simulink model "mu_t_2021b_temp"  (R2023b)
settings: Solver=VariableStepAuto  StartTime=0.0  StopTime=120  FixedStep=0.01  RelTol=1e-3
InitFcn:
  | %rho_0t=[0.29;0.29;0.29]; %m
  | %V_0t=[-0.001;-0.001;0];%[-0.0005;-0.0005;0];
  | %w_t=[0;0;-0.002];
  | 
  | 
  | %rho_0t=[0.3;0.3;0.2]; %m
  | %V_0t=[-0.001;-0.001;0];%[-0.0005;-0.0005;0];
  | %w_t=[0;0;-0.001];
values from neighbouring files (symbols this model uses):
  g_cm = zeros(4,4,n)    [Initiate_KUKA_inv.m]    (also in KUKA_Main.m)
  iota0 = eye(6,6)    [Initiate_KUKA_inv.m]    (also in KUKA_Main.m)
  K_d = 10*[1.3*eye(3) zeros(3);zeros(3) 0.8*eye(3)]    [Initiate_FQ.m]    (also in Initiate_KUKA_inv.m = 5*[0.7*eye(3) zeros(3);zeros(3) 0.5*eye(3)]; KUKA_Main.m = 50*[0.7*eye(3) zeros(3);zeros(3) 0.5*eye(3)])
  K_i = 5*[0.1*eye(3) zeros(3);zeros(3) 0.01*eye(3)]    [Initiate_FQ.m]    (also in Initiate_KUKA_inv.m = 5*[0.01*eye(3) zeros(3);zeros(3) 0.001*eye(3)]; KUKA_Main.m = 50*[0.01*eye(3) zeros(3);zeros(3) 0.001*eye(3)])
  K_p = 100*[0.1 0 0 0 0 0;0 0.1 0 0 0 0; 0 0 0.1 0 0 0; 0 0 0 0.01 0 0 ... (first row only)    [Initiate_FQ.m]    (also in Initiate_KUKA_inv.m = 5*[0.1 0 0 0 0 0;0 0.1 0 0 0 0; 0 0 0.1 0 0 0; 0 0 0 0.01 0 ; KUKA_Main.m = 50*[0.1 0 0 0 0 0;0 0.1 0 0 0 0; 0 0 0.1 0 0 0; 0 0 0 0.01 0)
  K_w = 200*eye(7)    [Initiate_FQ.m]
  K_wd = 2*eye(7)    [Initiate_FQ.m]
  M0 = M_temp.M0.data(:,:,1)    [Initiate_FQ.m]    (also in KUKA_Main.m)
  m0 = robot.Bodies{1,n+1}.Mass    [Initiate_KUKA_inv.m]    (also in KUKA_Main.m)
  m0_frak = diag_M(1:6,1:6)    [Initiate_KUKA_inv.m]
  M0m = M_temp.M0m.data(:,:,1)    [Initiate_FQ.m]    (also in KUKA_Main.m)
  m_diag = diag_M(7:end,7:end)    [Initiate_KUKA_inv.m]
  M_t = (((Adjoint(g_It))'\M_t_body)/(Adjoint(g_It)))    [Initiate_FQ.m]    (also in Initiate_KUKA_inv.m = [eye(3)*mt zeros(3); zeros(3) eye(3)*80]; KUKA_Main.m = [eye(3)*mt zeros(3); zeros(3) eye(3)*80])
  Mm = simplify(transpose(Xi_m)*transpose(Lm)*diagM*Lm*Xi_m)    [KUKA_Main.m]
  mm = zeros(1,n)    [Initiate_KUKA_inv.m]    (also in KUKA_Main.m)
  mu = P0    [Initiate_FQ.m]    (also in Initiate_KUKA_inv.m = zeros(6,1); KUKA_Main.m = P)
  mu_t = inv((Adjoint(g_It))')*M_t_body*[V_It;w_t]    [Initiate_FQ.m]    (also in Initiate_KUKA_inv.m = M_t*[V_0t;w_t]; KUKA_Main.m = M_t*[V_0t;w_t])
  q_dot_m = [0;0;0;0;0;0;0]    [Initiate_FQ.m]    (also in Initiate_KUKA_inv.m; KUKA_Main.m = [qdot1;qdot2;qdot3;qdot4;qdot5;qdot6;qdot7])
  q_m = [0.2;1.2;0.3;2.5;0.5;1.5;0.6]    [Initiate_FQ.m]    (also in Initiate_KUKA_inv.m = [0;0;0;0;0;0;0]; KUKA_Main.m = [q_m1;q_m2;q_m3;q_m4;q_m5;q_m6;q_m7])
  rho_It = [-0.3;-0.3;-0.1]    [Initiate_FQ.m]
  sc_size = 1    [Initiate_KUKA_inv.m]    (also in KUKA_Main.m)
  V_I0 = [-0.0001;-0.0001;0.0;-0.001;0.001;0.002]    [Initiate_FQ.m]    (also in Initiate_KUKA_inv.m = [0;0;0;0;0;0]; KUKA_Main.m = [0;0;0;0;0;0])
  V_It = 0.1.*[0.01;0.01;0]    [Initiate_FQ.m]
  Xi_m = Xi_m(1:robot.n*6,1:robot.n)    [KUKA_Main.m]
  Xi_m_matrix = zeros(6*n,n)    [Initiate_KUKA_inv.m]    (also in KUKA_Main.m)
undefined symbols (not defined in the file or in its folder): Dt, Dt_s, g_cm0, g_It00, I0, Ie, Im, me, noise_st, X, Y, Z
libraries: nesl_utility x195, sm_lib x180, robotcorelib x12, simulink x6
(part 7 of 8)

== system mu_t_2021b_temp/Space Manipulator4/join//link 1/iiwa_link_1 ==
  Inertia : sm_lib/Body Elements/Inertia  InertiaType=Custom  Mass=mm(6)  MassUnits=kg  CenterOfMass=[0, 0, 0]  CenterOfMassUnits=m  MomentsOfInertia=[Im(1,1,6) Im(2,2,6) Im(3,3,6)]  MomentsOfInertiaUnits=kg*m^2  ProductsOfInertia=[Im(3,2,6) Im(3,1,6) Im(2,1,6)]  ProductsOfInertiaUnits=kg*m^2  GraphicType=None  MarkerShape=Inertia  MarkerSize=20  GraphicVisPropType=SimpleVisualProperties  GraphicDiffuseColor=[0.5 0.5 0.5]  GraphicSpecularColor=[0.5 0.5 0.5 1.0]  GraphicAmbientColor=[0.15 0.15 0.15 1.0]  GraphicEmissiveColor=[0.0 0.0 0.0 1.0]  GraphicShininess=75  GraphicOpacity=1.0
  Visual : sm_lib/Body Elements/File Solid  ExtGeomFileName=iiwa_description/meshes/iiwa7/visual/link_1.stl  UnitType=Custom  ExtGeomFileUnits=m  StepReaderType=HEX  ExportConvexHullGeometry=off  InertiaType=Custom  Mass=0  MassUnits=kg  CenterOfMass=[0, 0, 0]  CenterOfMassUnits=m  MomentsOfInertia=[0, 0, 0]  MomentsOfInertiaUnits=kg*m^2  ProductsOfInertia=[0, 0, 0]  ProductsOfInertiaUnits=kg*m^2  BasedOnType=DensityFromFile  Density=1000  DensityUnits=kg/m^3  DoExposeReferenceFrame=on  SerializedFrames=<Frames/>  GraphicType=FromGeometry  MarkerShape=Sphere  MarkerSize=10  GraphicVisPropType=SimpleVisualProperties  GraphicDiffuseColor=[1, 0.423529411765, 0.0392156862745]  GraphicSpecularColor=[0.5 0.5 0.5 1.0]  GraphicAmbientColor=[0.15 0.15 0.15 1.0]  GraphicEmissiveColor=[0.0 0.0 0.0 1.0]  GraphicShininess=75  GraphicOpacity=1
  VisualOriginTransform : sm_lib/Frames and Transforms/Rigid Transform  TranslationMethod=Cartesian  TranslationStandardOffset=0  TranslationStandardOffsetUnits=m  TranslationStandardAxis=+Z  TranslationCartesianOffset=[0, 0, 0]  TranslationCartesianOffsetUnits=m  TranslationROffset=0  TranslationROffsetUnits=m  TranslationZOffset=0  TranslationZOffsetUnits=m  TranslationThetaOffset=0  TranslationThetaOffsetUnits=deg  RotationMethod=RotationSequence  RotationAngleUnits=deg  RotationStandardAxis=+Z  RotationAngle=0.0  RotationArbitraryAxis=[0 0 1]  FollAlignAxisA=+X  BaseAlignAxisA=+Y  FollAlignAxisB=+Y  BaseAlignAxisB=+Z  RotationSequenceAxes=BaseAxes  RotationSequence=XYZ  RotationSequenceAngles=[0, 0, 0]  RotationSequenceAnglesUnits=rad  RotationMatrix=[1 0 0; 0 1 0; 0 0 1]  Quaternion=[1 0 0 0]
  iiwa_joint_2_OriginTransform : sm_lib/Frames and Transforms/Rigid Transform  TranslationMethod=Cartesian  TranslationStandardOffset=0  TranslationStandardOffsetUnits=m  TranslationStandardAxis=+Z  TranslationCartesianOffset=g_cm(1:3,4,6)'  TranslationCartesianOffsetUnits=m  TranslationROffset=0  TranslationROffsetUnits=m  TranslationZOffset=0  TranslationZOffsetUnits=m  TranslationThetaOffset=0  TranslationThetaOffsetUnits=deg  RotationMethod=RotationMatrix  RotationAngleUnits=deg  RotationStandardAxis=+Z  RotationAngle=0.0  RotationArbitraryAxis=[0 0 1]  FollAlignAxisA=+X  BaseAlignAxisA=+Y  FollAlignAxisB=+Y  BaseAlignAxisB=+Z  RotationSequenceAxes=BaseAxes  RotationSequence=XYZ  RotationSequenceAngles=[1.57079632679, 0, 3.14159265359]  RotationSequenceAnglesUnits=rad  RotationMatrix=g_cm(1:3,1:3,6)  Quaternion=[1 0 0 0]
  F : PMIOPort  Side=Left
  F1 : PMIOPort  Port=2  Side=Right
  connections:
  Visual/RConn1 -- VisualOriginTransform/RConn1
  VisualOriginTransform/LConn1 -- Inertia/RConn1 -- iiwa_joint_2_OriginTransform/RConn1 -- F/RConn1
  F1/RConn1 -- iiwa_joint_2_OriginTransform/LConn1

== system mu_t_2021b_temp/Space Manipulator4/joint//link2/iiwa_link_2 ==
  Inertia : sm_lib/Body Elements/Inertia  InertiaType=Custom  Mass=mm(5)  MassUnits=kg  CenterOfMass=[0, 0, 0]  CenterOfMassUnits=m  MomentsOfInertia=[Im(1,1,5) Im(2,2,5) Im(3,3,5)]  MomentsOfInertiaUnits=kg*m^2  ProductsOfInertia=[Im(3,2,5) Im(3,1,5) Im(2,1,5)]  ProductsOfInertiaUnits=kg*m^2  GraphicType=None  MarkerShape=Inertia  MarkerSize=20  GraphicVisPropType=SimpleVisualProperties  GraphicDiffuseColor=[0.5 0.5 0.5]  GraphicSpecularColor=[0.5 0.5 0.5 1.0]  GraphicAmbientColor=[0.15 0.15 0.15 1.0]  GraphicEmissiveColor=[0.0 0.0 0.0 1.0]  GraphicShininess=75  GraphicOpacity=1.0
  Visual : sm_lib/Body Elements/File Solid  ExtGeomFileName=iiwa_description/meshes/iiwa7/visual/link_2.stl  UnitType=Custom  ExtGeomFileUnits=m  StepReaderType=HEX  ExportConvexHullGeometry=off  InertiaType=Custom  Mass=0  MassUnits=kg  CenterOfMass=[0, 0, 0]  CenterOfMassUnits=m  MomentsOfInertia=[0, 0, 0]  MomentsOfInertiaUnits=kg*m^2  ProductsOfInertia=[0, 0, 0]  ProductsOfInertiaUnits=kg*m^2  BasedOnType=DensityFromFile  Density=1000  DensityUnits=kg/m^3  DoExposeReferenceFrame=on  SerializedFrames=<Frames/>  GraphicType=FromGeometry  MarkerShape=Sphere  MarkerSize=10  GraphicVisPropType=SimpleVisualProperties  GraphicDiffuseColor=[1, 0.423529411765, 0.0392156862745]  GraphicSpecularColor=[0.5 0.5 0.5 1.0]  GraphicAmbientColor=[0.15 0.15 0.15 1.0]  GraphicEmissiveColor=[0.0 0.0 0.0 1.0]  GraphicShininess=75  GraphicOpacity=1
  VisualOriginTransform : sm_lib/Frames and Transforms/Rigid Transform  TranslationMethod=Cartesian  TranslationStandardOffset=0  TranslationStandardOffsetUnits=m  TranslationStandardAxis=+Z  TranslationCartesianOffset=[0, 0, 0]  TranslationCartesianOffsetUnits=m  TranslationROffset=0  TranslationROffsetUnits=m  TranslationZOffset=0  TranslationZOffsetUnits=m  TranslationThetaOffset=0  TranslationThetaOffsetUnits=deg  RotationMethod=RotationSequence  RotationAngleUnits=deg  RotationStandardAxis=+Z  RotationAngle=0.0  RotationArbitraryAxis=[0 0 1]  FollAlignAxisA=+X  BaseAlignAxisA=+Y  FollAlignAxisB=+Y  BaseAlignAxisB=+Z  RotationSequenceAxes=BaseAxes  RotationSequence=XYZ  RotationSequenceAngles=[0, 0, 0]  RotationSequenceAnglesUnits=rad  RotationMatrix=[1 0 0; 0 1 0; 0 0 1]  Quaternion=[1 0 0 0]
  iiwa_joint_3_OriginTransform : sm_lib/Frames and Transforms/Rigid Transform  TranslationMethod=Cartesian  TranslationStandardOffset=0  TranslationStandardOffsetUnits=m  TranslationStandardAxis=+Z  TranslationCartesianOffset=g_cm(1:3,4,5)'  TranslationCartesianOffsetUnits=m  TranslationROffset=0  TranslationROffsetUnits=m  TranslationZOffset=0  TranslationZOffsetUnits=m  TranslationThetaOffset=0  TranslationThetaOffsetUnits=deg  RotationMethod=RotationMatrix  RotationAngleUnits=deg  RotationStandardAxis=+Z  RotationAngle=0.0  RotationArbitraryAxis=[0 0 1]  FollAlignAxisA=+X  BaseAlignAxisA=+Y  FollAlignAxisB=+Y  BaseAlignAxisB=+Z  RotationSequenceAxes=BaseAxes  RotationSequence=XYZ  RotationSequenceAngles=[1.57079632679, 0, 3.14159265359]  RotationSequenceAnglesUnits=rad  RotationMatrix=g_cm(1:3,1:3,5)  Quaternion=[1 0 0 0]
  F : PMIOPort  Side=Left
  F1 : PMIOPort  Port=2  Side=Right
  connections:
  Visual/RConn1 -- VisualOriginTransform/RConn1
  VisualOriginTransform/LConn1 -- Inertia/RConn1 -- iiwa_joint_3_OriginTransform/RConn1 -- F/RConn1
  iiwa_joint_3_OriginTransform/LConn1 -- F1/RConn1

== system mu_t_2021b_temp/Space Manipulator4/joint//link3/iiwa_link_3 ==
  Inertia : sm_lib/Body Elements/Inertia  InertiaType=Custom  Mass=mm(4)  MassUnits=kg  CenterOfMass=[0, 0, 0]  CenterOfMassUnits=m  MomentsOfInertia=[Im(1,1,4) Im(2,2,4) Im(3,3,4)]  MomentsOfInertiaUnits=kg*m^2  ProductsOfInertia=[Im(3,2,4) Im(3,1,4) Im(2,1,4)]  ProductsOfInertiaUnits=kg*m^2  GraphicType=None  MarkerShape=Inertia  MarkerSize=20  GraphicVisPropType=SimpleVisualProperties  GraphicDiffuseColor=[0.5 0.5 0.5]  GraphicSpecularColor=[0.5 0.5 0.5 1.0]  GraphicAmbientColor=[0.15 0.15 0.15 1.0]  GraphicEmissiveColor=[0.0 0.0 0.0 1.0]  GraphicShininess=75  GraphicOpacity=1.0
  Visual : sm_lib/Body Elements/File Solid  ExtGeomFileName=iiwa_description/meshes/iiwa7/visual/link_3.stl  UnitType=Custom  ExtGeomFileUnits=m  StepReaderType=HEX  ExportConvexHullGeometry=off  InertiaType=Custom  Mass=0  MassUnits=kg  CenterOfMass=[0, 0, 0]  CenterOfMassUnits=m  MomentsOfInertia=[0, 0, 0]  MomentsOfInertiaUnits=kg*m^2  ProductsOfInertia=[0, 0, 0]  ProductsOfInertiaUnits=kg*m^2  BasedOnType=DensityFromFile  Density=1000  DensityUnits=kg/m^3  DoExposeReferenceFrame=on  SerializedFrames=<Frames/>  GraphicType=FromGeometry  MarkerShape=Sphere  MarkerSize=10  GraphicVisPropType=SimpleVisualProperties  GraphicDiffuseColor=[1, 0.423529411765, 0.0392156862745]  GraphicSpecularColor=[0.5 0.5 0.5 1.0]  GraphicAmbientColor=[0.15 0.15 0.15 1.0]  GraphicEmissiveColor=[0.0 0.0 0.0 1.0]  GraphicShininess=75  GraphicOpacity=1
  VisualOriginTransform : sm_lib/Frames and Transforms/Rigid Transform  TranslationMethod=Cartesian  TranslationStandardOffset=0  TranslationStandardOffsetUnits=m  TranslationStandardAxis=+Z  TranslationCartesianOffset=[0, 0, -0.026]  TranslationCartesianOffsetUnits=m  TranslationROffset=0  TranslationROffsetUnits=m  TranslationZOffset=0  TranslationZOffsetUnits=m  TranslationThetaOffset=0  TranslationThetaOffsetUnits=deg  RotationMethod=RotationSequence  RotationAngleUnits=deg  RotationStandardAxis=+Z  RotationAngle=0.0  RotationArbitraryAxis=[0 0 1]  FollAlignAxisA=+X  BaseAlignAxisA=+Y  FollAlignAxisB=+Y  BaseAlignAxisB=+Z  RotationSequenceAxes=BaseAxes  RotationSequence=XYZ  RotationSequenceAngles=[0, 0, 0]  RotationSequenceAnglesUnits=rad  RotationMatrix=[1 0 0; 0 1 0; 0 0 1]  Quaternion=[1 0 0 0]
  iiwa_joint_4_OriginTransform : sm_lib/Frames and Transforms/Rigid Transform  TranslationMethod=Cartesian  TranslationStandardOffset=0  TranslationStandardOffsetUnits=m  TranslationStandardAxis=+Z  TranslationCartesianOffset=g_cm(1:3,4,4)'  TranslationCartesianOffsetUnits=m  TranslationROffset=0  TranslationROffsetUnits=m  TranslationZOffset=0  TranslationZOffsetUnits=m  TranslationThetaOffset=0  TranslationThetaOffsetUnits=deg  RotationMethod=RotationMatrix  RotationAngleUnits=deg  RotationStandardAxis=+Z  RotationAngle=0.0  RotationArbitraryAxis=[0 0 1]  FollAlignAxisA=+X  BaseAlignAxisA=+Y  FollAlignAxisB=+Y  BaseAlignAxisB=+Z  RotationSequenceAxes=BaseAxes  RotationSequence=XYZ  RotationSequenceAngles=[1.57079632679, 0, 0]  RotationSequenceAnglesUnits=rad  RotationMatrix=g_cm(1:3,1:3,4)  Quaternion=[1 0 0 0]
  F : PMIOPort  Side=Left
  F1 : PMIOPort  Port=2  Side=Right
  connections:
  VisualOriginTransform/LConn1 -- iiwa_joint_4_OriginTransform/RConn1 -- Inertia/RConn1 -- F/RConn1
  Visual/RConn1 -- VisualOriginTransform/RConn1
  iiwa_joint_4_OriginTransform/LConn1 -- F1/RConn1

== system mu_t_2021b_temp/Space Manipulator4/joint//link4/iiwa_link_4 ==
  Inertia : sm_lib/Body Elements/Inertia  InertiaType=Custom  Mass=mm(3)  MassUnits=kg  CenterOfMass=[0, 0, 0]  CenterOfMassUnits=m  MomentsOfInertia=[Im(1,1,3) Im(2,2,3) Im(3,3,3)]  MomentsOfInertiaUnits=kg*m^2  ProductsOfInertia=[Im(3,2,3) Im(3,1,3) Im(2,1,3)]  ProductsOfInertiaUnits=kg*m^2  GraphicType=None  MarkerShape=Inertia  MarkerSize=20  GraphicVisPropType=SimpleVisualProperties  GraphicDiffuseColor=[0.5 0.5 0.5]  GraphicSpecularColor=[0.5 0.5 0.5 1.0]  GraphicAmbientColor=[0.15 0.15 0.15 1.0]  GraphicEmissiveColor=[0.0 0.0 0.0 1.0]  GraphicShininess=75  GraphicOpacity=1.0
  Visual : sm_lib/Body Elements/File Solid  ExtGeomFileName=iiwa_description/meshes/iiwa7/visual/link_4.stl  UnitType=Custom  ExtGeomFileUnits=m  StepReaderType=HEX  ExportConvexHullGeometry=off  InertiaType=Custom  Mass=0  MassUnits=kg  CenterOfMass=[0, 0, 0]  CenterOfMassUnits=m  MomentsOfInertia=[0, 0, 0]  MomentsOfInertiaUnits=kg*m^2  ProductsOfInertia=[0, 0, 0]  ProductsOfInertiaUnits=kg*m^2  BasedOnType=DensityFromFile  Density=1000  DensityUnits=kg/m^3  DoExposeReferenceFrame=on  SerializedFrames=<Frames/>  GraphicType=FromGeometry  MarkerShape=Sphere  MarkerSize=10  GraphicVisPropType=SimpleVisualProperties  GraphicDiffuseColor=[1, 0.423529411765, 0.0392156862745]  GraphicSpecularColor=[0.5 0.5 0.5 1.0]  GraphicAmbientColor=[0.15 0.15 0.15 1.0]  GraphicEmissiveColor=[0.0 0.0 0.0 1.0]  GraphicShininess=75  GraphicOpacity=1
  VisualOriginTransform : sm_lib/Frames and Transforms/Rigid Transform  TranslationMethod=Cartesian  TranslationStandardOffset=0  TranslationStandardOffsetUnits=m  TranslationStandardAxis=+Z  TranslationCartesianOffset=[0, 0, 0]  TranslationCartesianOffsetUnits=m  TranslationROffset=0  TranslationROffsetUnits=m  TranslationZOffset=0  TranslationZOffsetUnits=m  TranslationThetaOffset=0  TranslationThetaOffsetUnits=deg  RotationMethod=RotationSequence  RotationAngleUnits=deg  RotationStandardAxis=+Z  RotationAngle=0.0  RotationArbitraryAxis=[0 0 1]  FollAlignAxisA=+X  BaseAlignAxisA=+Y  FollAlignAxisB=+Y  BaseAlignAxisB=+Z  RotationSequenceAxes=BaseAxes  RotationSequence=XYZ  RotationSequenceAngles=[0, 0, 0]  RotationSequenceAnglesUnits=rad  RotationMatrix=[1 0 0; 0 1 0; 0 0 1]  Quaternion=[1 0 0 0]
  iiwa_joint_5_OriginTransform : sm_lib/Frames and Transforms/Rigid Transform  TranslationMethod=Cartesian  TranslationStandardOffset=0  TranslationStandardOffsetUnits=m  TranslationStandardAxis=+Z  TranslationCartesianOffset=g_cm(1:3,4,3)'  TranslationCartesianOffsetUnits=m  TranslationROffset=0  TranslationROffsetUnits=m  TranslationZOffset=0  TranslationZOffsetUnits=m  TranslationThetaOffset=0  TranslationThetaOffsetUnits=deg  RotationMethod=RotationMatrix  RotationAngleUnits=deg  RotationStandardAxis=+Z  RotationAngle=0.0  RotationArbitraryAxis=[0 0 1]  FollAlignAxisA=+X  BaseAlignAxisA=+Y  FollAlignAxisB=+Y  BaseAlignAxisB=+Z  RotationSequenceAxes=BaseAxes  RotationSequence=XYZ  RotationSequenceAngles=[-1.57079632679, 3.14159265359, 0]  RotationSequenceAnglesUnits=rad  RotationMatrix=g_cm(1:3,1:3,3)  Quaternion=[1 0 0 0]
  F : PMIOPort  Side=Left
  F1 : PMIOPort  Port=2  Side=Right
  connections:
  Visual/RConn1 -- VisualOriginTransform/RConn1
  VisualOriginTransform/LConn1 -- Inertia/RConn1 -- iiwa_joint_5_OriginTransform/RConn1 -- F/RConn1
  iiwa_joint_5_OriginTransform/LConn1 -- F1/RConn1

== system mu_t_2021b_temp/Space Manipulator4/joint//link5/iiwa_link_5 ==
  Inertia : sm_lib/Body Elements/Inertia  InertiaType=Custom  Mass=mm(2)  MassUnits=kg  CenterOfMass=[0, 0, 0]  CenterOfMassUnits=m  MomentsOfInertia=[Im(1,1,2) Im(2,2,2) Im(3,3,2)]  MomentsOfInertiaUnits=kg*m^2  ProductsOfInertia=[Im(3,2,2) Im(3,1,2) Im(2,1,2)]  ProductsOfInertiaUnits=kg*m^2  GraphicType=None  MarkerShape=Inertia  MarkerSize=20  GraphicVisPropType=SimpleVisualProperties  GraphicDiffuseColor=[0.5 0.5 0.5]  GraphicSpecularColor=[0.5 0.5 0.5 1.0]  GraphicAmbientColor=[0.15 0.15 0.15 1.0]  GraphicEmissiveColor=[0.0 0.0 0.0 1.0]  GraphicShininess=75  GraphicOpacity=1.0
  Visual : sm_lib/Body Elements/File Solid  ExtGeomFileName=iiwa_description/meshes/iiwa7/visual/link_5.stl  UnitType=Custom  ExtGeomFileUnits=m  StepReaderType=HEX  ExportConvexHullGeometry=off  InertiaType=Custom  Mass=0  MassUnits=kg  CenterOfMass=[0, 0, 0]  CenterOfMassUnits=m  MomentsOfInertia=[0, 0, 0]  MomentsOfInertiaUnits=kg*m^2  ProductsOfInertia=[0, 0, 0]  ProductsOfInertiaUnits=kg*m^2  BasedOnType=DensityFromFile  Density=1000  DensityUnits=kg/m^3  DoExposeReferenceFrame=on  SerializedFrames=<Frames/>  GraphicType=FromGeometry  MarkerShape=Sphere  MarkerSize=10  GraphicVisPropType=SimpleVisualProperties  GraphicDiffuseColor=[1, 0.423529411765, 0.0392156862745]  GraphicSpecularColor=[0.5 0.5 0.5 1.0]  GraphicAmbientColor=[0.15 0.15 0.15 1.0]  GraphicEmissiveColor=[0.0 0.0 0.0 1.0]  GraphicShininess=75  GraphicOpacity=1
  VisualOriginTransform : sm_lib/Frames and Transforms/Rigid Transform  TranslationMethod=Cartesian  TranslationStandardOffset=0  TranslationStandardOffsetUnits=m  TranslationStandardAxis=+Z  TranslationCartesianOffset=[0, 0, -0.026]  TranslationCartesianOffsetUnits=m  TranslationROffset=0  TranslationROffsetUnits=m  TranslationZOffset=0  TranslationZOffsetUnits=m  TranslationThetaOffset=0  TranslationThetaOffsetUnits=deg  RotationMethod=RotationSequence  RotationAngleUnits=deg  RotationStandardAxis=+Z  RotationAngle=0.0  RotationArbitraryAxis=[0 0 1]  FollAlignAxisA=+X  BaseAlignAxisA=+Y  FollAlignAxisB=+Y  BaseAlignAxisB=+Z  RotationSequenceAxes=BaseAxes  RotationSequence=XYZ  RotationSequenceAngles=[0, 0, 0]  RotationSequenceAnglesUnits=rad  RotationMatrix=[1 0 0; 0 1 0; 0 0 1]  Quaternion=[1 0 0 0]
  iiwa_joint_6_OriginTransform : sm_lib/Frames and Transforms/Rigid Transform  Commented=on  TranslationMethod=Cartesian  TranslationStandardOffset=0  TranslationStandardOffsetUnits=m  TranslationStandardAxis=+Z  TranslationCartesianOffset=[0, 0.0607 , 0.19]  TranslationCartesianOffsetUnits=m  TranslationROffset=0  TranslationROffsetUnits=m  TranslationZOffset=0  TranslationZOffsetUnits=m  TranslationThetaOffset=0  TranslationThetaOffsetUnits=deg  RotationMethod=RotationSequence  RotationAngleUnits=deg  RotationStandardAxis=+Z  RotationAngle=0.0  RotationArbitraryAxis=[0 0 1]  FollAlignAxisA=+X  BaseAlignAxisA=+Y  FollAlignAxisB=+Y  BaseAlignAxisB=+Z  RotationSequenceAxes=BaseAxes  RotationSequence=XYZ  RotationSequenceAngles=[1.57079632679, 0, 0]  RotationSequenceAnglesUnits=rad  RotationMatrix=[1 0 0; 0 1 0; 0 0 1]  Quaternion=[1 0 0 0]
  iiwa_joint_6_OriginTransform1 : sm_lib/Frames and Transforms/Rigid Transform  TranslationMethod=Cartesian  TranslationStandardOffset=0  TranslationStandardOffsetUnits=m  TranslationStandardAxis=+Z  TranslationCartesianOffset=g_cm(1:3,4,2)'  TranslationCartesianOffsetUnits=m  TranslationROffset=0  TranslationROffsetUnits=m  TranslationZOffset=0  TranslationZOffsetUnits=m  TranslationThetaOffset=0  TranslationThetaOffsetUnits=deg  RotationMethod=RotationMatrix  RotationAngleUnits=deg  RotationStandardAxis=+Z  RotationAngle=0.0  RotationArbitraryAxis=[0 0 1]  FollAlignAxisA=+X  BaseAlignAxisA=+Y  FollAlignAxisB=+Y  BaseAlignAxisB=+Z  RotationSequenceAxes=BaseAxes  RotationSequence=XYZ  RotationSequenceAngles=[1.57079632679, 0, 0]  RotationSequenceAnglesUnits=rad  RotationMatrix=g_cm(1:3,1:3,2)  Quaternion=[1 0 0 0]
  F : PMIOPort  Side=Left
  F1 : PMIOPort  Port=2  Side=Right
  connections:
  Visual/RConn1 -- VisualOriginTransform/RConn1
  iiwa_joint_6_OriginTransform1/RConn1 -- Inertia/RConn1 -- VisualOriginTransform/LConn1 -- F/RConn1
  iiwa_joint_6_OriginTransform1/LConn1 -- F1/RConn1

== system mu_t_2021b_temp/Space Manipulator4/joint//link6/iiwa_link_6 ==
  Inertia : sm_lib/Body Elements/Inertia  InertiaType=Custom  Mass=mm(1)  MassUnits=kg  CenterOfMass=[0, 0, 0]  CenterOfMassUnits=m  MomentsOfInertia=[Im(1,1,1) Im(2,2,1) Im(3,3,1)]  MomentsOfInertiaUnits=kg*m^2  ProductsOfInertia=[Im(3,2,1) Im(3,1,1) Im(2,1,1)]  ProductsOfInertiaUnits=kg*m^2  GraphicType=None  MarkerShape=Inertia  MarkerSize=20  GraphicVisPropType=SimpleVisualProperties  GraphicDiffuseColor=[0.5 0.5 0.5]  GraphicSpecularColor=[0.5 0.5 0.5 1.0]  GraphicAmbientColor=[0.15 0.15 0.15 1.0]  GraphicEmissiveColor=[0.0 0.0 0.0 1.0]  GraphicShininess=75  GraphicOpacity=1.0
  Visual : sm_lib/Body Elements/File Solid  ExtGeomFileName=iiwa_description/meshes/iiwa7/visual/link_6.stl  UnitType=Custom  ExtGeomFileUnits=m  StepReaderType=HEX  ExportConvexHullGeometry=off  InertiaType=Custom  Mass=0  MassUnits=kg  CenterOfMass=[0, 0, 0]  CenterOfMassUnits=m  MomentsOfInertia=[0, 0, 0]  MomentsOfInertiaUnits=kg*m^2  ProductsOfInertia=[0, 0, 0]  ProductsOfInertiaUnits=kg*m^2  BasedOnType=DensityFromFile  Density=1000  DensityUnits=kg/m^3  DoExposeReferenceFrame=on  SerializedFrames=<Frames/>  GraphicType=FromGeometry  MarkerShape=Sphere  MarkerSize=10  GraphicVisPropType=SimpleVisualProperties  GraphicDiffuseColor=[1, 0.423529411765, 0.0392156862745]  GraphicSpecularColor=[0.5 0.5 0.5 1.0]  GraphicAmbientColor=[0.15 0.15 0.15 1.0]  GraphicEmissiveColor=[0.0 0.0 0.0 1.0]  GraphicShininess=75  GraphicOpacity=1
  VisualOriginTransform : sm_lib/Frames and Transforms/Rigid Transform  TranslationMethod=Cartesian  TranslationStandardOffset=0  TranslationStandardOffsetUnits=m  TranslationStandardAxis=+Z  TranslationCartesianOffset=[0, 0, 0.0607 ]  TranslationCartesianOffsetUnits=m  TranslationROffset=0  TranslationROffsetUnits=m  TranslationZOffset=0  TranslationZOffsetUnits=m  TranslationThetaOffset=0  TranslationThetaOffsetUnits=deg  RotationMethod=RotationSequence  RotationAngleUnits=deg  RotationStandardAxis=+Z  RotationAngle=0.0  RotationArbitraryAxis=[0 0 1]  FollAlignAxisA=+X  BaseAlignAxisA=+Y  FollAlignAxisB=+Y  BaseAlignAxisB=+Z  RotationSequenceAxes=BaseAxes  RotationSequence=XYZ  RotationSequenceAngles=[0, 0, 0]  RotationSequenceAnglesUnits=rad  RotationMatrix=[1 0 0; 0 1 0; 0 0 1]  Quaternion=[1 0 0 0]
  iiwa_joint_7_OriginTransform : sm_lib/Frames and Transforms/Rigid Transform  TranslationMethod=Cartesian  TranslationStandardOffset=0  TranslationStandardOffsetUnits=m  TranslationStandardAxis=+Z  TranslationCartesianOffset=g_cm(1:3,4,1)'  TranslationCartesianOffsetUnits=m  TranslationROffset=0  TranslationROffsetUnits=m  TranslationZOffset=0  TranslationZOffsetUnits=m  TranslationThetaOffset=0  TranslationThetaOffsetUnits=deg  RotationMethod=RotationMatrix  RotationAngleUnits=deg  RotationStandardAxis=+Z  RotationAngle=0.0  RotationArbitraryAxis=[0 0 1]  FollAlignAxisA=+X  BaseAlignAxisA=+Y  FollAlignAxisB=+Y  BaseAlignAxisB=+Z  RotationSequenceAxes=BaseAxes  RotationSequence=XYZ  RotationSequenceAngles=[-1.57079632679, 3.14159265359, 0]  RotationSequenceAnglesUnits=rad  RotationMatrix=g_cm(1:3,1:3,1)  Quaternion=[1 0 0 0]
  F : PMIOPort  Side=Left
  F1 : PMIOPort  Port=2  Side=Right
  connections:
  iiwa_joint_7_OriginTransform/RConn1 -- Inertia/RConn1 -- F/RConn1 -- VisualOriginTransform/LConn1
  Visual/RConn1 -- VisualOriginTransform/RConn1
  iiwa_joint_7_OriginTransform/LConn1 -- F1/RConn1

== system mu_t_2021b_temp/Space Manipulator4/joint//link7/iiwa_link_7 ==
  Inertia : sm_lib/Body Elements/Inertia  InertiaType=Custom  Mass=m0  MassUnits=kg  CenterOfMass=[0, 0, 0]  CenterOfMassUnits=m  MomentsOfInertia=[I0(1,1) I0(2,2) I0(3,3)]  MomentsOfInertiaUnits=kg*m^2  ProductsOfInertia=[I0(3,2) I0(3,1) I0(2,1)]  ProductsOfInertiaUnits=kg*m^2  GraphicType=None  MarkerShape=Inertia  MarkerSize=20  GraphicVisPropType=SimpleVisualProperties  GraphicDiffuseColor=[0.5 0.5 0.5]  GraphicSpecularColor=[0.5 0.5 0.5 1.0]  GraphicAmbientColor=[0.15 0.15 0.15 1.0]  GraphicEmissiveColor=[0.0 0.0 0.0 1.0]  GraphicShininess=75  GraphicOpacity=1.0
  Visual : sm_lib/Body Elements/File Solid  ExtGeomFileName=iiwa_description/meshes/iiwa7/visual/link_7.stl  UnitType=Custom  ExtGeomFileUnits=m  StepReaderType=HEX  ExportConvexHullGeometry=off  InertiaType=Custom  Mass=0  MassUnits=kg  CenterOfMass=[0, 0, 0]  CenterOfMassUnits=m  MomentsOfInertia=[0, 0, 0]  MomentsOfInertiaUnits=kg*m^2  ProductsOfInertia=[0, 0, 0]  ProductsOfInertiaUnits=kg*m^2  BasedOnType=DensityFromFile  Density=1000  DensityUnits=kg/m^3  DoExposeReferenceFrame=on  SerializedFrames=<Frames/>  GraphicType=FromGeometry  MarkerShape=Sphere  MarkerSize=10  GraphicVisPropType=SimpleVisualProperties  GraphicDiffuseColor=[0.4, 0.4, 0.4]  GraphicSpecularColor=[0.5 0.5 0.5 1.0]  GraphicAmbientColor=[0.15 0.15 0.15 1.0]  GraphicEmissiveColor=[0.0 0.0 0.0 1.0]  GraphicShininess=75  GraphicOpacity=1
  VisualOriginTransform : sm_lib/Frames and Transforms/Rigid Transform  TranslationMethod=Cartesian  TranslationStandardOffset=0  TranslationStandardOffsetUnits=m  TranslationStandardAxis=+Z  TranslationCartesianOffset=[0, 0, 0]  TranslationCartesianOffsetUnits=m  TranslationROffset=0  TranslationROffsetUnits=m  TranslationZOffset=0  TranslationZOffsetUnits=m  TranslationThetaOffset=0  TranslationThetaOffsetUnits=deg  RotationMethod=RotationSequence  RotationAngleUnits=deg  RotationStandardAxis=+Z  RotationAngle=0.0  RotationArbitraryAxis=[0 0 1]  FollAlignAxisA=+X  BaseAlignAxisA=+Y  FollAlignAxisB=+Y  BaseAlignAxisB=+Z  RotationSequenceAxes=BaseAxes  RotationSequence=XYZ  RotationSequenceAngles=[0, 0, 0]  RotationSequenceAnglesUnits=rad  RotationMatrix=[1 0 0; 0 1 0; 0 0 1]  Quaternion=[1 0 0 0]
  iiwa_joint_ee_OriginTransform : sm_lib/Frames and Transforms/Rigid Transform  TranslationMethod=Cartesian  TranslationStandardOffset=0  TranslationStandardOffsetUnits=m  TranslationStandardAxis=+Z  TranslationCartesianOffset=g_cm0(1:3,4)'  TranslationCartesianOffsetUnits=m  TranslationROffset=0  TranslationROffsetUnits=m  TranslationZOffset=0  TranslationZOffsetUnits=m  TranslationThetaOffset=0  TranslationThetaOffsetUnits=deg  RotationMethod=RotationMatrix  RotationAngleUnits=deg  RotationStandardAxis=+Z  RotationAngle=0.0  RotationArbitraryAxis=[0 0 1]  FollAlignAxisA=+X  BaseAlignAxisA=+Y  FollAlignAxisB=+Y  BaseAlignAxisB=+Z  RotationSequenceAxes=BaseAxes  RotationSequence=XYZ  RotationSequenceAngles=[0, 0, 0]  RotationSequenceAnglesUnits=rad  RotationMatrix=g_cm0(1:3,1:3)  Quaternion=[1 0 0 0]
  F : PMIOPort  Side=Left
  F1 : PMIOPort  Port=2  Side=Right
  connections:
  F/RConn1 -- iiwa_joint_ee_OriginTransform/RConn1 -- VisualOriginTransform/LConn1 -- Inertia/RConn1
  Visual/RConn1 -- VisualOriginTransform/RConn1
  iiwa_joint_ee_OriginTransform/LConn1 -- F1/RConn1

== matlab function mu_t_2021b_temp/Controller/nullspace_mapping ==
  data: Mm input; K_w_grad_w input; q_dot_m input; Z input; Z_dagger input; f_N output; Z_dot_dagger input; K_nu_nu input; f_pot input; out2 output; fw_i input
function [f_N, out2] =null_space(Mm, K_w_grad_w, q_dot_m,Z, Z_dagger,Z_dot_dagger, K_nu_nu, f_pot, fw_i)

f_N=zeros(7,1);

% nu=Z_dagger*q_dot_m;


f_N=Mm*Z*(-Z_dot_dagger*q_dot_m-K_nu_nu-Z_dagger*K_w_grad_w-0.01.*fw_i +100.*Z_dagger*f_pot);

out2=Z_dagger*K_w_grad_w;

% 
% for i=1:m
%     fw =fw+ dot(w_opt, null_space(:,i)) / norm(null_space(:,i))^2 * null_space(:,i);
% end

% for i=1:m
%     fw =fw+ dot(f_pot, null_space(:,i)) / norm(null_space(:,i))^2 * null_space(:,i);
% end

% A_dot=A_partial*q_dot;


% JJ=A/Mm;
% null_space=eye(7)-(JJ'/(JJ*JJ'))*JJ;
% fw=zeros(7,1);
% fw=fw+null_space*f_pot;
% f_N=fw+null_space*w_opt;

== matlab function mu_t_2021b_temp/Controller/grad w ==
  data: A input; grad_w output; A_partial input; q_dot input
function grad_w  = grad_w(A,A_partial, q_dot)

w=sqrt(det(A*A'));

n=length(q_dot);
grad_w=zeros(n,1);
for i=1:n
    grad_w(i) = w/2* trace(   (A*A')\(A*A_partial(:,:,i)'+A_partial(:,:,i)*A')    );%det(A*A')*trace(inv(A')A_dot'+inv(A')*inv(A)*A_dot*A');
end

% w_dot=1/norm(grad_w'*q_dot);

== matlab function mu_t_2021b_temp/Dynamic Parameters/V_I1 ==
  data: P input; A_connection input; q_dot_m input; M0 input; V_I0 output; g_I0 input
function V_I0 = V_I0(P, A_connection, q_dot_m, M0, g_I0)
V_I0=Adjoint(g_I0)*((M0\P)-A_connection*q_dot_m);

== matlab function mu_t_2021b_temp/Controller/Velocity_error1 ==
  data: w input; out output; in input
function out = cut_off(w, in)

if w<0.003
    out=0.*in; %adjoint_low(Adjoint(g_I0)*V_Ie)*Adjoint(inv(g_I0))*V_It+Adjoint(inv(g_I0))*V_It_dot
else
    out=in;
end

== matlab function mu_t_2021b_temp/Controller/Potential Function1 ==
  data: w_p output; p_0n input
function w_p = norm( p_0n)

w_p=norm(p_0n);

== matlab function mu_t_2021b_temp/Space Manipulator4/collect positions ==
  data: p_joints output; p_02 input; p_03 input; p_04 input; p_05 input
function p_joints = collect_positions(p_02,p_03,p_04,p_05)

% p_joints=zeros(3,5);
p_joints=[p_02 p_03 p_04 p_05];

== matlab function mu_t_2021b_temp/Controller/joint distance from spacecraft ==
  data: pnorm output; p_joints input
function pnorm = norm( p_joints)

pnorm=zeros(4,1);
for i=1:4
    pnorm(i)=norm(p_joints(:,i));
end

== matlab function mu_t_2021b_temp/Controller/Potential Function3 ==
  data: f_pot output; p_joints input; g_n0 input; sc_size input; A input
function f_pot = potential_joints( p_joints, g_n0, sc_size, A)

w_joints=zeros(1,4);
grad_w_joints=zeros(3,4);
grad_w_jointspace=zeros(7,4);
f_pot=zeros(7,1);
gain=0.02.*[70 70 70 70];

J_joints=zeros(4,6,7);
for i=1:4
    J_joints(i,:,:)=Adjoint(inv(g_n0))*[A(:,1:i+1) 0.*A(:,i+2:end)];
end


temp=zeros(6,7);
    for i=1:4 %------------------------------ Joints collision w Spacecraft
        w_joints(i)=norm(p_joints(:,i));%+[0; 0; 0.15]);
        grad_w_joints(:,i)=-(p_joints(:,i))/(w_joints(i)^3);
        temp(:,:)=J_joints(i,:,:);
        grad_w_jointspace(:,i)=temp'*[grad_w_joints(:,i);zeros(3,1)];
        if w_joints(i)<sqrt(2)*sc_size/2
            f_pot=f_pot-((1/(1+100*exp(1000*(w_joints(i)-(sqrt(2)*sc_size/2+0.05)))))*gain(i)*(-grad_w_jointspace(:,i))); 
        end
    end

== matlab function mu_t_2021b_temp/Space Manipulator4/collect positions1 ==
  data: g_joints output; g_02 input; g_03 input; g_04 input; g_05 input
function g_joints = collect_poses(g_02,g_03,g_04,g_05)

g_joints=zeros(4,4,4);
% p_joints=zeros(3,5);
g_joints(1,:,:)=g_02;
g_joints(2,:,:)=g_03;
g_joints(3,:,:)=g_04;
g_joints(4,:,:)=g_05;

== matlab function mu_t_2021b_temp/Controller/Z dagger derivative ==
  data: Z_dagger input; N_dot input; Z_dot_dagger output; Z_dot input
function Z_dot_dagger =Z_dot_dagger(Z_dagger,N_dot,Z_dot)

Z_dot_dagger=Z_dagger*N_dot-Z_dagger*Z_dot*Z_dagger;

== matlab function mu_t_2021b_temp/Controller/Nullspace derivatives ==
  data: Mm input; A input; N_dot output; Mm_partial input; A_partial input; q_dot input; Z_dot output; j input; Nj input
function [N_dot,Z_dot] =Nullspace_derivatives(Mm,A,Mm_partial,A_partial,q_dot,j, Nj)

Mm_dot=zeros(7);
A_dot=zeros(6,7);
for i=1:length(Mm_partial(1,1,:))
    Mm_dot=Mm_dot+Mm_partial(:,:,i).*q_dot(i);
    A_dot=A_dot+A_partial(:,:,i).*q_dot(i);
end

%parts of N_dot

N1=((Mm\Mm_dot)/Mm)     *   A'   / ((A/Mm)*A')*A;
N2=-Mm\A_dot'   /   ((A/Mm)*A')   * A;
N3=(Mm\A')   /   ((A/Mm)*A')    * ((A_dot/Mm)*A'  -   (A/Mm) *(Mm_dot /Mm) *A'    +   (A/Mm)*A_dot') /   ((A/Mm)*A')   *   A;
N4=-(Mm\ A') *    ((A/Mm)*A')  *A_dot;

N_dot=N1+N2+N3+N4;

% Z_dot=N_dot(:,j);%/norm_Z;
Nj_dot=N_dot(:,j);

Z_dot=Nj_dot/norm(Nj)-Nj'*Nj_dot*Nj/norm(Nj)^3;

== matlab function mu_t_2021b_temp/Controller/Z ==
  data: N input; Z output; Z_dagger output; Mm input; j output; Nj output
function [Z,Z_dagger,j,Nj] =Z(N,Mm)

% m=length(temp(1,:));
% 
% for i=1:m
%     Z(:,i)=Mm*temp(:,i);
% end
nN=zeros(7,1);
for j=1:7
    nN(j,1)=N(:,j)'*N(:,j);
end

[nmax,j]=max(nN);

Z=N(:,j)/norm(N(:,j));

Z_dagger=(Z'*Mm*Z)\(Z'*Mm);

norm_Z=norm(N(:,j));

Nj=N(:,j);

== matlab function mu_t_2021b_temp/Dynamic Parameters/MATLAB Function1 ==
  data: g_I0 input; mu input; P output
function P=Momentum(g_I0,mu)
% find the momentum in current base frame
P=Adjoint(g_I0)'*mu;

== matlab function mu_t_2021b_temp/Controller/Nullspace_maps ==
  data: Mm input; A input; N output; q_dot_m input
function N  =Nullspace_maps(Mm,A,q_dot_m)

n=length(q_dot_m);

N_Am=eye(n)-(Mm\A') *   (   (   (A/Mm) *   A')\    A);
N=N_Am;

== matlab function mu_t_2021b_temp/Controller/ZKw ==
  data: Z_dagger input; K_w_grad_w input; out output
function out  =for_i(Z_dagger, K_w_grad_w)


out=Z_dagger*K_w_grad_w;

== matlab function mu_t_2021b_temp/Controller/sensing noise in g_t ==
  data: err input; errM output
function errM = fcn(err)

errM=expm(wedge(err));

== matlab function mu_t_2021b_temp/Controller/Kinematics/velocity of target in EE ==
  data: g_te input; V_It_e output; V_It input
function V_It_e = V_It(g_te,V_It)
% Eq 25, second half
V_It_e=Adjoint(inv(g_te))*V_It;

== matlab function mu_t_2021b_temp/Controller/V_It_2 ==
  data: mu_t input; M_t_body input; g_It input; V_It_2 output
function V_It_2 = V_It(mu_t, M_t_body, g_It)


% g_gpt=[eye(3) [0.25; 0.25; 0.25]; 0 0 0 1];
R=g_It(1:3,1:3);

% Pt=(Adjoint(g_It))'*mu_t;
V_It_2=(Adjoint(g_It))*inv(M_t_body)*(Adjoint(g_It)')*mu_t;%(Mt\(Adjoint(g_It)')*Pt); %[R zeros(3);zeros(3) R]


% Ad g_Igp(t) M^-1 Ad gI_gp(t)' inv(Ad g_I_gp') Mt inv (Ad g_I_gp) V_Igp

== matlab function mu_t_2021b_temp/Controller/Potential Function ==
  data: U_ff output; A input; w input; grad_w input; U_c input; p_0n input; p_joints input; sc_size input; Mm_hat input
function U_ff = U_ff(A,w,grad_w, U_c, p_0n, p_joints, sc_size,Mm_hat)

w_p=norm(p_0n);
grad_w_p=-p_0n/((w_p)^3); % d/dt(1/sqrt(x^2+y^2+z^2)) = -1/2*w_p^3 * d/dt (x^2+...)
w_lim=0.002;
% w_joints=zeros(1,4);
% grad_w_joints=zeros(3,4);
% 
%     for i=1:4 %------------------------------ Joints collision w Spacecraft
%         w_joints(i)=norm(p_joints(:,i));
%         grad_w_joints(:,i)=-p_joints(:,i)/(w_joints(i)^3);
%         if w_joints(i)<sqrt(2)*sc_size/2+0.05
%             U_c=U_c-[(1/(1+100*exp(1000*(w_joints(i)-(sqrt(2)*sc_size/2+0.05)))))*1*(-grad_w_joints(:,i)); zeros(3,1)]; 
%         end
%     end

JJ=A;
A_dagger = ((Mm_hat)\JJ')/((JJ/Mm_hat)*JJ');

if w<w_lim %--------------------------------------------- close to singular
%     temp=(pinv(A)'*grad_w);
%     dir=(temp)./(norm(temp));
%     Uc=U_c-dot(U_c,dir).*dir;

    if w_p<sqrt(2)*sc_size/2+0.0 %-------------- EE collision w Spacecraft
        U_c=U_c-[(1/(1+100*exp(1000*(w_p-(sqrt(2)*sc_size/2+0.05)))))*0.5*(-grad_w_p); zeros(3,1)]; 
    end
    
    U_ff=U_c-(1*(1-w_lim/w)*(w_lim/w^2).*A_dagger'*grad_w);%(1/(1+100*exp(1000*(w-0.003))))*0.0001*pinv(A)'*(-grad_w./(w^2)); 
    %adjoint_low(Adjoint(g_I0)*V_Ie)*Adjoint(inv(g_I0))*V_It+Adjoint(inv(g_I0))*V_It_dot

else %----------------------------------------------- NOT close to singular
    
    if w_p<sqrt(2)*sc_size/2+0.0 %-------------- EE collision w Spacecraft
        U_c=U_c-[(1/(1+100*exp(1000*(w_p-(sqrt(2)*sc_size/2+0.05)))))*0.5*(-grad_w_p); zeros(3,1)]; 
    end

    U_ff=U_c;
end

== matlab function mu_t_2021b_temp/Inverse Dynamics/C_hat1/AMA_partial ==
  data: q_m input; AMA_partial output; M0 input; A input; A_partial input; V input; M0_partial input
function AMA_partial = AMA_partial(q_m,M0,A,A_partial,V,M0_partial)
% Calculates the C_hat_m matrix from base pose and arm joint angles

n=length(q_m);
b=length(V);

% find the temp intermediate term
AMA_partial=zeros(n,n,n);
for i=1:n
    AMA_partial(1:n,1:n,i)=transpose(A_partial(1:end,1:end,i))*M0*A+transpose(A)*M0_partial(1:end,1:end,i)*A+transpose(A)*M0*A_partial(1:end,1:end,i); %calcualte the derivative of not-augmented arm mass matrix from equation 121 of TRO paper
end

== matlab function mu_t_2021b_temp/Inverse Dynamics/C_hat1/A_partial ==
  data: q_m input; A_partial output; M0 input; M0_partial input; M0m_partial input; M0m input; V input
function A_partial = A_partial(q_m,M0,M0_partial,M0m_partial,M0m,V)
% Calculates the C_hat_m matrix from base pose and arm joint angles

n=length(q_m);
b=length(V);

% Find partial of connection A to each joint angle
A_partial=zeros(b,n,n);

temp1=zeros(b,n);
temp2=zeros(b,n);
temp3=zeros(b,n);

for i=1:n
    temp1=M0\M0_partial(1:end,1:end,i);
    temp2=M0\M0m;
    temp3=M0\M0m_partial(1:end,1:end,i);
    A_partial(1:b,1:n,i)=-temp1*temp2+temp3; % Equation 122
end

== matlab function mu_t_2021b_temp/Controller/mu_init ==
  data: g_It input; Mt input; V_It input; mu_t output
function mu_t = mu_init(g_It,Mt,V_It)

R_It=g_It(1:3,1:3);
V_Itb=[R_It' zeros(3);zeros(3) R_It']*V_It;

mu_t=Adjoint(g_It)'\ Mt*V_Itb;
% mu_init=Mt*V_It; %*(inv(Adjoint(g_It)))


% Ad g_Igp(t) M^-1 Ad gI_gp(t)' inv(Ad g_I_gp') Mt inv (Ad g_I_gp) V_Igp

== matlab function mu_t_2021b_temp/Controller/sensing noise in g_t1 ==
  data: z input; errM output; z_gt input
function errM = fcn(z,z_gt)

g_te=(z\z_gt);

R_te=g_te(1:3,1:3);
p_te=g_te(1:3,4);

temp_R=eye(3)-R_te;
temp_R=0.5*trace(temp_R);

temp_p=0.5*transpose(p_te)*p_te;
errM =temp_R+temp_p;

== matlab function mu_t_2021b_temp/Controller/Triggered Subsystem/MATLAB Function ==
  data: Z input; X_pos_out output double; Dt input; Mass_matrix input; X_pos input; mu_vector input; P_pos input; Q input; R input; P_pos_out output double
function [X_pos_out,P_pos_out] = fcn(Z,Dt,Mass_matrix,X_pos,mu_vector,P_pos,Q,R)
% X_pos_out=eye(4);
% P_pos_out=zeros(6);
mu_vector = [mu_vector(4:6);mu_vector(1:3)];

Omega = Dt*inv(Mass_matrix)*Adjoint_EKF(inv(X_pos))*mu_vector;
D   = DMatrix(X_pos,Dt,Mass_matrix,mu_vector);
F   = Adjoint_EKF(expm(wedge_EKF(-Omega)))...
                   +Right_Jacob_SE(Omega)*D; 
X_pri = X_pos*expm(wedge_EKF(Omega));
P_pri = F*P_pos*F'...
                   +Right_Jacob_SE(Omega)*Q*Right_Jacob_SE(Omega)';
nu        = LieAlgebra(inv(h_fcn(X_pri))*Z);
H = [1 0 0 0 0 0; 0 1 0 0 0 0; 0 0 1 0 0 0; 0 0 0 1 0 0;0 0 0 0 1 0;0 0 0 0 0 1];
K     = P_pri*H'*inv(H*P_pri*H'+R);
X_pos_out = X_pri*real(expm(wedge_EKF( K*nu))) ;
P_pos_out = real(Right_Jacob_SE(K*nu)*(eye(6)-K*H)...
                   *P_pri*Right_Jacob_SE(K*nu)');

== matlab function mu_t_2021b_temp/Controller/sensing noise in g_t2 ==
  data: z input; errM output; z_gt input
function errM = fcn(z,z_gt)

g_te=(z\z_gt);

R_te=g_te(1:3,1:3);
p_te=g_te(1:3,4);

temp_R=eye(3)-R_te;
temp_R=0.5*trace(temp_R);

temp_p=0.5*transpose(p_te)*p_te;
errM =temp_R+temp_p;

== matlab function mu_t_2021b_temp/Dynamic Parameters/ 1 ==
  data: q_m input; L0 output; Lm0 output; Lm output; Xi_m input
function [L0,Lm0,Lm] =L_calculator(q_m,Xi_m)
% Calculates the time-dependent L matrix
n=length(q_m);
L=zeros(6*(n+1),6*(n+1));
% Compute M_frak for ith body
% Calculate L matrix
for i=1:n+1
    for j=1:n+1
        if i>j
            Ad_temp=eye(6);
            for k=j:i-1
                Ad_temp=Adjoint(g_Matrix(-Xi_m(:,k),q_m(k)))*Ad_temp;
            end
            L(6*(i-1)+1:6*(i-1)+6,6*(j-1)+1:6*(j-1)+6)=Ad_temp;
        elseif i==j
            L(6*(i-1)+1:6*(i-1)+6,6*(j-1)+1:6*(j-1)+6)=eye(6);
        elseif i<j
            L(6*(i-1)+1:6*(i-1)+6,6*(j-1)+1:6*(j-1)+6)=zeros(6);
        end
    end
end

L0=L(1:6,1:6);
Lm0=L(7:end,1:6);
Lm=L(7:end,7:end);

end

== matlab function mu_t_2021b_temp/Inverse Dynamics/C_hat1/C_hat ==
  data: q_m input; Mm_hat_partial input; q_dot_m input; C_hat output
function C_hat = C_hat(q_m, Mm_hat_partial,q_dot_m)
% Calculates the C_hat_m matrix from base pose and arm joint angles

n=length(q_m);


% Calculate C_hat matrix
C_temp1=zeros(n,n);
C_temp2=zeros(n,n);
C_hat=zeros(n,n);
for i=1:n
    C_temp1=C_temp1+squeeze(Mm_hat_partial(1:n,1:n,i)).*q_dot_m(i); % nxn by scalar
    C_temp2(i,1:n)=0.5*transpose(q_dot_m)*squeeze(Mm_hat_partial(1:n,1:n,i)); %1xn by nxn 
end

C_hat=C_temp1-C_temp2;

== matlab function mu_t_2021b_temp/Inverse Dynamics/C_hat1/Lm_partials/Lm0partial ==
  data: q_m input; Lm0_partial output; Xi_m input; iota0 input
function Lm0_partial = Lm0_partial(q_m,Xi_m,iota0)
% Calculates the C_hat_m matrix from base pose and arm joint angles

n=length(q_m);

% Find partial of Lm to joint angles
Lm0_partial=zeros(6*n,6,n); % 6nx6xn
for i=1:n
    for j=1:n
        Lm0_partial(6*(j-1)+1:6*j,1:6,i)=Ad_partial(j,1,i,Xi_m,q_m,iota0); % equation 114 of TRO paper
    end
end

%%%%%%%%%%%%%%%%%%%%%%%%%%%%%%%%%%%%%%%%%%%%%%%%%%%%%%%%%%%%% MUST BE
%%%%%%%%%%%%%%%%%%%%%%%%%%%%%%%%%%%%%%%%%%%%%%%%%%%%%%%%%%%%% CHECKED

== matlab function mu_t_2021b_temp/Inverse Dynamics/C_hat1/Lm_partials/Lmpartial ==
  data: q_m input; Lm_partial output; Xi_m input; iota0 input
function Lm_partial  = Lm_partial(q_m,Xi_m,iota0)
% Calculates the C_hat_m matrix from base pose and arm joint angles

n=length(q_m);

% Find partial of Lm0 to joint angles
Lm_partial=zeros(6*n,6*n,n); % 6nx6xn
for i=1:n
    Lm_partial(:,:,i)=zeros(6*n,6*n);
    for j=2:n
        for k=2:n
            if j>i && i>=k
                Lm_partial(6*(j-1)+1:6*j,6*(k-2)+1:6*(k-1),i)=Ad_partial(j,k,i,Xi_m,q_m,iota0); % equation 81 of TRO paper
            elseif i==j && i>=k
                Lm_partial(6*(j-1)+1:6*j,6*(k-2)+1:6*(k-1),i)=Ad_partial(j,k,i,Xi_m,q_m,iota0); % equation 81 of TRO paper
            else
                Lm_partial(6*(j-1)+1:6*(j-1)+6,6*(k-2)+1:6*(k-2)+6,i)=zeros(6,6);
            end

        end
    end
end

== matlab function mu_t_2021b_temp/Inverse Dynamics/C_hat1/M_partials/ M0partial ==
  data: q_m input; M0_partial output; Lm0 input; V input; iota0 input; diag_Mm input; Lm0_partial input
function M0_partial = M0_partial(q_m,Lm0,V,iota0,diag_Mm,Lm0_partial)
% Calculates the C_hat_m matrix from base pose and arm joint angles

n=length(q_m);
b=length(V);

% Find partial of M0 to joint angles
M0_partial=zeros(b,b,n); %initiate
for i=1:n
    temp1=transpose(Lm0_partial(1:end,1:end,i))*diag_Mm*Lm0;
    temp2=transpose(Lm0)*diag_Mm*Lm0_partial(1:end,1:end,i);
    M0_partial(1:b,1:b,i)= iota0'*(temp1+temp2)*iota0; %6x6 %equation 117 of TRO
end

== matlab function mu_t_2021b_temp/Inverse Dynamics/C_hat1/M_partials/M0mpartial ==
  data: q_m input; M0m_partial output; V input; Lm input; Lm0 input; iota0 input; diag_Mm input; Lm0_partial input; Lm_partial input; Xi_m_matrix input
function M0m_partial = M0m_partial(q_m,V,Lm,Lm0,iota0,diag_Mm,Lm0_partial,Lm_partial, Xi_m_matrix)
% Calculates the C_hat_m matrix from base pose and arm joint angles

n=length(q_m);
b=length(V);

% Find partial of M0m to joint angles
M0m_partial=zeros(b,n,n);
for i=1:n
    temp1=transpose(Lm0_partial(1:end,1:end,i))*diag_Mm*Lm;
    temp2=transpose(Lm0)*diag_Mm*Lm_partial(1:end,1:end,i);
    M0m_partial(1:b,1:n,i)= iota0'*(temp1+temp2)*Xi_m_matrix; % equation 118 of TRO paper
end

== matlab function mu_t_2021b_temp/Inverse Dynamics/C_hat1/M_partials/Mmpartial ==
  data: q_m input; Mm_partial output; Xi_m_matrix input; Lm input; diag_Mm input; Lm_partial input
function Mm_partial = Mm_partial(q_m,Xi_m_matrix,Lm,diag_Mm,Lm_partial)
% Calculates the C_hat_m matrix from base pose and arm joint angles

n=length(q_m);

% find the non-generalized arm mass matrix'x derivative to joint angles
Mm_partial=zeros(n,n,n);
for i=1:n
    temp=   transpose(Lm_partial(1:6*n,1:6*n,i))*diag_Mm*Lm  +   transpose(Lm)*diag_Mm*Lm_partial(1:6*n,1:6*n,i);
    Mm_partial(1:n,1:n,i)=transpose(Xi_m_matrix)*temp*Xi_m_matrix; %calcualte the derivative of not-augmented arm mass matrix from equation 120 of TRO paper
end

== matlab function mu_t_2021b_temp/Controller/gradient_of_Eg ==
  data: g_te input; Nabla_Eg output
function Nabla_Eg = fcn(g_te)

% Calculate the gradient of the Pose Error Function
p_te=g_te(1:3,4);
R_te=g_te(1:3,1:3);

temp=0.5*(R_te-transpose(R_te));

R_temp=vee3(temp);

Nabla_Eg=[p_te;R_temp];

== matlab function mu_t_2021b_temp/Inverse Dynamics/C_hat1/Mm_hat_partial ==
  data: q_m input; AMA_partial input; Mm_hat_partial output; Mm_partial input
function Mm_hat_partial = Mm_hat_partial(q_m, AMA_partial, Mm_partial)
% Calculates the C_hat_m matrix from base pose and arm joint angles

n=length(q_m);

% find the generalized arm mass matrix'x derivative to joint angles
Mm_hat_partial=zeros(n,n,n);
for i=1:n
    Mm_hat_partial(1:n,1:n,i)=Mm_partial(1:n,1:n,i)-AMA_partial(1:n,1:n,i); %calcualte the derivative of augmented arm mass matrix from equation 119 of TRO paper
end

== matlab function mu_t_2021b_temp/Inverse Dynamics/N_hat1/N_hat ==
  data: N_hat_temp output; q_m input; q_dot_m input; A input; V input; P input; M0_partial input; A_partial input; iota0 input; M0 input
function N_hat_temp = N_hat(q_m,q_dot_m,A,V,P,M0_partial, A_partial, iota0, M0)
% Calculates the N_hat_m matrix from base pose and arm joint angles

n=length(q_m);
b=length(V);

%Form N_hat from equation 19 of ACC paper
N_temp1=zeros(n,b); N_temp2=zeros(n,b); N_temp3=zeros(n,b);

for i=1:n
    N_temp1=N_temp1+transpose(squeeze(A_partial(1:b,1:n,i)).*q_dot_m(i)); % transpose of (bxn times 1x1) 
    N_temp2(i,1:b)=transpose(q_dot_m)*transpose(squeeze(A_partial(1:b,1:n,i))); %1xn times nxb
    N_temp3(i,1:b)=0.5*transpose(P)*(M0\M0_partial(1:end,1:end,i))*inv(M0); % 1xb times bxb
end

N_hat_temp=transpose(A)*transpose(adjoint_low(V,iota0))-N_temp1+N_temp2+N_temp3;

== matlab function mu_t_2021b_temp/Space Manipulator2/Q2q ==
  data: Q input; qm output
function qm = Q2q(Q)

qm=quat2eul(Q','XYZ')';

== matlab function mu_t_2021b_temp/Space Manipulator2/Q2q1 ==
  data: Q input; qm output
function qm = Q2q(Q)

qm=quat2eul(Q','XYZ')';

== matlab function mu_t_2021b_temp/Inverse Dynamics/A_dot ==
  data: A_partial input; q_m_dot input; A_dot output
function A_dot = fcn(A_partial, q_m_dot)
n=length(q_m_dot);

A_dot=zeros(6,n);
for i=1:n
    A_dot=A_dot+A_partial(:,:,i).*q_m_dot(i);
end

== matlab function mu_t_2021b_temp/Inverse Dynamics/C_hat/AMA_partial ==
  data: q_m input; AMA_partial output; M0 input; A input; A_partial input; V input; M0_partial input
function AMA_partial = AMA_partial(q_m,M0,A,A_partial,V,M0_partial)
% Calculates the C_hat_m matrix from base pose and arm joint angles

n=length(q_m);
b=length(V);

% find the temp intermediate term
AMA_partial=zeros(n,n,n);
for i=1:n
    AMA_partial(1:n,1:n,i)=transpose(A_partial(1:end,1:end,i))*M0*A+transpose(A)*M0_partial(1:end,1:end,i)*A+transpose(A)*M0*A_partial(1:end,1:end,i); %calcualte the derivative of not-augmented arm mass matrix from equation 121 of TRO paper
end

== matlab function mu_t_2021b_temp/Inverse Dynamics/C_hat/A_partial ==
  data: q_m input; A_partial output; M0 input; M0_partial input; M0m_partial input; M0m input; V input
function A_partial = A_partial(q_m,M0,M0_partial,M0m_partial,M0m,V)
% Calculates the C_hat_m matrix from base pose and arm joint angles

n=length(q_m);
b=length(V);

% Find partial of connection A to each joint angle
A_partial=zeros(b,n,n);

temp1=zeros(b,n);
temp2=zeros(b,n);
temp3=zeros(b,n);

for i=1:n
    temp1=M0\(M0_partial(:,:,i));
    temp2=M0\M0m;
    temp3=M0\(M0m_partial(:,:,i));
    A_partial(1:b,1:n,i)=-temp1*temp2+temp3; % Equation 122
end

== matlab function mu_t_2021b_temp/Controller/Kinematics/g_te ==
  data: g_Ie input; g_It input; g_te output
function g_te = relative_pose(g_Ie, g_It)
% Calculates the relative pose of end-effector to target from the absolute
% poses of the end-effector and the target
g_te = inverse(g_It)*g_Ie;

== matlab function mu_t_2021b_temp/Inverse Dynamics/C_hat/C_hat1 ==
  data: q_m input; Mm_hat_partial input; q_dot_m input; C_hat output
function C_hat = C_hat(q_m, Mm_hat_partial,q_dot_m)
% Calculates the C_hat_m matrix from base pose and arm joint angles

n=length(q_m);


% Calculate C_hat matrix
C_temp1=zeros(n,n);
C_temp2=zeros(n,n);
C_hat=zeros(n,n);
for i=1:n
    C_temp1=C_temp1+squeeze(Mm_hat_partial(1:n,1:n,i)).*q_dot_m(i); % nxn by scalar
    C_temp2(i,1:n)=0.5*transpose(q_dot_m)*squeeze(Mm_hat_partial(1:n,1:n,i)); %1xn by nxn 
end

C_hat=C_temp1-C_temp2;

== matlab function mu_t_2021b_temp/Inverse Dynamics/C_hat/Lm_partials/Lm0partial ==
  data: q_m input; Lm0_partial output; Xi_m input; iota0 input
function Lm0_partial = Lm0_partial(q_m,Xi_m,iota0)
% Calculates the C_hat_m matrix from base pose and arm joint angles

n=length(q_m);

% Find partial of Lm to joint angles
Lm0_partial=zeros(6*n,6,n); % 6nx6xn
for i=1:n
    for j=1:n
        Lm0_partial(6*(j-1)+1:6*j,1:6,i)=Ad_partial(j,1,i,Xi_m,q_m,iota0); % equation 114 of TRO paper
    end
end

%%%%%%%%%%%%%%%%%%%%%%%%%%%%%%%%%%%%%%%%%%%%%%%%%%%%%%%%%%%%% MUST BE
%%%%%%%%%%%%%%%%%%%%%%%%%%%%%%%%%%%%%%%%%%%%%%%%%%%%%%%%%%%%% CHECKED
